simulink model "ATI_NetFT_nano43_PC104"  (R2016a)
settings: Solver=ode3  StartTime=0.0  StopTime=inf  FixedStep=dt  RelTol=1e-3
InitFcn:
  | PSMCMD_DEPENDENCY
  | init_NetFt
  | init_scopes
  | init_udp
  | init_resolved_rates
  | ATI_Init_nano43
  | init_LinIntPathPlan
  | init_force_control
undefined symbols (not defined in the file or in its folder): A, ATI_torque_convert_to_Nmm, filter_coeffs_ATI, filter_coeffs_bias, inv_T, N_ATI, N_bias
libraries: dspswit3 x1, xpcsensoraylib x1, xpcobsoletelib x1, xpcrtudplib x1, slrtlib x1
settings Model: Creator=Andrea  LastModifiedBy=Rashid
settings SolverCC: EnableConcurrentExecution=on
settings DataIOCC: LimitDataPoints=on  SaveFormat=Array  SignalLoggingSaveFormat=ModelDataLogs
settings OptimizationCC: BlockReduction=off  OptimizeBlockIOStorage=off  BufferReuse=off  GlobalBufferReuse=off  ExpressionFolding=off  ExpressionDepthLimit=2147483647  LocalBlockOutputs=off  OptimizeModelRefInitCode=on
settings DebuggingCC: UnderspecifiedInitializationDetection=Classic  MergeDetectMultiDrivingBlocksExec=none  SolverPrmCheckMsg=warning  MultiTaskCondExecSysMsg=warning  MultiTaskRateTransMsg=warning  FcnCallInpInsideContextMsg=UseLocalSettings  StateNameClashWarn=warning
settings HardwareCC: ProdBitPerPointer=32  ProdLargestAtomicFloat=None  ProdWordSize=32  ProdLongLongMode=on  ProdHWDeviceType=Generic->32-bit x86 compatible
settings ModelReferenceCC: PropagateSignalLabelsOutOfModel=off
settings SFSimCC: SimParseCustomCode=off
settings RTWCC: SystemTargetFile=slrtert.tlc  TLCOptions=-aSLRTFTZOFF=1  TemplateMakefile=slrtert_default_tmf  Description=Simulink Real-Time (ERT)  RTWCompilerOptimization=Custom  RTWCustomCompilerOptimizations=/arch=IA32
settings CodeAppCC: CustomSymbolStrType=$N$R$M  InternalIdentifier=Classic
settings SimulinkRealTimeERTCC: TargetFcnLib=ansi_tfl_table_tmw.mat  GenFloatMathFcnCalls=NOT IN USE  TargetLangStandard=C89/C90 (ANSI)  CodeReplacementLibrary=XPC_BLAS  UtilityFuncGeneration=Auto  ERTMultiwordTypeDef=System defined  ERTMultiwordLength=256  MultiwordLength=2048  GenerateFullHeader=on  InferredTypesCompatibility=off  GenerateSampleERTMain=off  GenerateTestInterfaces=off  ModelReferenceCompliant=on  ParMdlRefBuildCompliant=on  CompOptLevelCompliant=on  ConcurrentExecutionCompliant=on  IncludeMdlTerminateFcn=on  GeneratePreprocessorConditionals=Disable all  CombineOutputUpdateFcns=off  CombineSignalStateStructs=off  SuppressErrorStatus=off  ERTFirstTimeCompliant=off  IncludeFileDelimiter=Auto  ERTCustomFileBanners=off  SupportAbsoluteTime=on  LogVarNameModifier=rt_  MatFileLogging=on  MultiInstanceERTCode=off  CodeInterfacePackaging=Nonreusable function  SupportNonFinite=on  SupportComplex=on  PurelyIntegerCode=off  SupportContinuousTime=on  SupportNonInlinedSFcns=on  SupportVariableSizeSignals=off  ParenthesesLevel=Nominal  CastingMode=Nominal  MATLABClassNameForMDSCustomization=xpcAperiodicCustomization  ModelStepFunctionPrototypeControlCompliant=off  CPPClassGenCompliant=off  AutosarCompliant=off  GRTInterface=on  GenerateAllocFcn=off  UseToolchainInfoCompliant=off  GenerateSharedConstants=on  ExtModeTransport=0  ExtModeStaticAlloc=off  ExtModeStaticAllocSize=1000000  ExtModeTesting=off  InlinedParameterPlacement=Hierarchical  TargetOS=BareBoardExample  MultiInstanceErrorCode=Error  RateGroupingCode=on  RootIOFormat=Individual arguments  RTWCAPIRootIO=off  EnableDataOwnership=off  ERTFilePackagingFormat=Modular  PreserveExpressionOrder=off  PreserveIfCondition=off  ConvertIfToSwitch=off  PreserveExternInFcnDecls=on  SuppressUnreachableDefaultCases=off  EnableSignedLeftShifts=on  EnableSignedRightShifts=on  IndentStyle=K&R  IndentSize=2  EnableUserReplacementTypes=off  MaxIdInt32=MAX_int32_T  MinIdInt32=MIN_int32_T  MaxIdUint32=MAX_uint32_T  MaxIdInt16=MAX_int16_T  MinIdInt16=MIN_int16_T  MaxIdUint16=MAX_uint16_T  MaxIdInt8=MAX_int8_T  MinIdInt8=MIN_int8_T  MaxIdUint8=MAX_uint8_T  BooleanTrueId=true  BooleanFalseId=false  MemSecPackage=--- None ---  MemSecDataConstants=Default  MemSecDataIO=Default  MemSecDataInternal=Default  MemSecDataParameters=Default  MemSecFuncInitTerm=Default  MemSecFuncExecute=Default  MemSecFuncSharedUtil=Default  GlobalDataDefinition=Auto  GlobalDataReference=Auto  GenerateASAP2=off  ERTSrcFileBannerTemplate=ert_code_template.cgt  ERTHdrFileBannerTemplate=ert_code_template.cgt  ERTDataSrcFileTemplate=ert_code_template.cgt  ERTDataHdrFileTemplate=ert_code_template.cgt  ERTCustomFileTemplate=example_file_process.tlc  SignalDisplayLevel=10  ParamTuneLevel=10  InitialValueSource=Model  RTWCAPISignals=off  RTWCAPIParams=on  RTWCAPIStates=off  RL32ModeModifier=Real-Time  ExtMode=on  ExtModeMexFile=ext_xpc  ExtModeIntrfLevel=Level2 - Open  ExtModeArmWhenConnect=off  RL32LogTETModifier=on  RL32LogBufSizeModifier=100000  xPCTaskExecutionProfile=off  xPCRL32EventNumber=5000  RL32IRQSourceModifier=Timer  xPCIRQSourceBoard=None/Other  xPCIOIRQSlot=-1  xpcObjCom=off  xPCGenerateASAP2=off  xPCGenerateXML=off  RL32ObjectName=tg  xPCisDownloadable=off  xPCisDefaultEnv=on  xPCisModelTimeout=on  xPCModelTimeoutSecs=5  xpcDblBuff=off  xPCLoadParamSetFile=off  xPCConcurrentTasks=off  xPCEnableSFAnimation=off
settings ConfigComp: CovModelRefEnable=Off

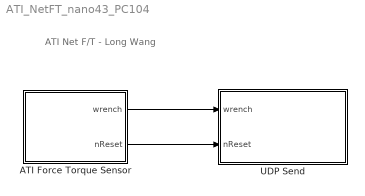
== system ATI_NetFT_nano43_PC104 ==
  note: ATI Net F/T - Long Wang
  ATI Force Torque Sensor : Subsystem
  UDP Send : Subsystem
  wires:
  ATI Force Torque Sensor/1(wrench) -> UDP Send/1(wrench)
  ATI Force Torque Sensor/2(nReset) -> UDP Send/2(nReset)

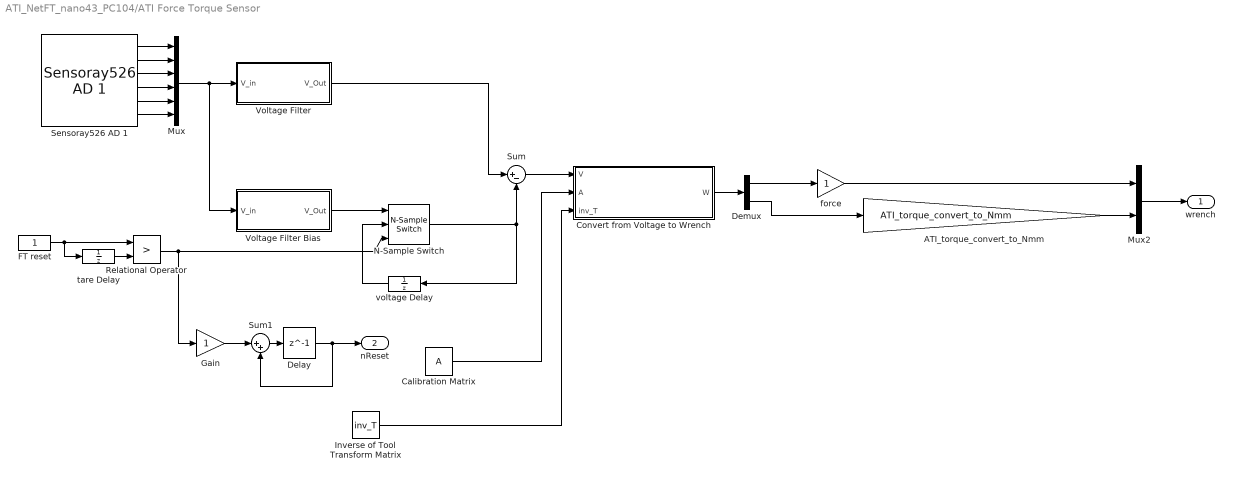
== system ATI_NetFT_nano43_PC104/ATI Force Torque Sensor ==
  ATI_torque_convert_to_Nmm : Gain  Gain=ATI_torque_convert_to_Nmm
  Calibration Matrix : Constant  Value=A
  "Convert from Voltage to Wrench " : MATLAB Function  TreatAsAtomicUnit=on
  Delay : Delay  DelayLength=1  InitialCondition=0
  Demux : Demux  Outputs=2
  FT reset : Constant
  Gain : Gain  OutDataTypeStr=double
  Inverse of Tool Transform Matrix : Constant  Value=inv_T  VectorParams1D=off
  Mux : Mux  Inputs=6
  Mux2 : Mux  Inputs=2
  N-Sample Switch : dspswit3/N-Sample Switch  N=3000  reset=on  TriggerType=Rising edge  Ts=-1
  Relational Operator : RelationalOperator  Operator=>  OutDataTypeStr=boolean
  Sensoray526 AD 1 : xpcsensoraylib/A//D/Sensoray526 AD 1  channel=[1 2 3 4 5 6]  sampletime=.002  baseaddress1=0x2c0  baseaddress2=0
  Sum : Sum  Inputs=|+-
  Sum1 : Sum  Inputs=|++
  Voltage Filter : Subsystem
  Voltage Filter Bias : Subsystem
  force : Gain
  tare Delay : UnitDelay  SampleTime=-1
  voltage Delay : UnitDelay  InitialCondition=zeros(6,1)  SampleTime=-1
  wrench : Outport
  nReset : Outport  Port=2
  wires:
  Sensoray526 AD 1/1 -> Mux/1
  Sensoray526 AD 1/2 -> Mux/2
  Sensoray526 AD 1/3 -> Mux/3
  Sensoray526 AD 1/4 -> Mux/4
  Sensoray526 AD 1/5 -> Mux/5
  Sensoray526 AD 1/6 -> Mux/6
  Calibration Matrix/1 -> "Convert from Voltage to Wrench "/2(A)
  Inverse of Tool Transform Matrix/1 -> "Convert from Voltage to Wrench "/3(inv_T)
  Sum/1 -> "Convert from Voltage to Wrench "/1(V)
  Voltage Filter/1(V_Out) -> Sum/1
  Demux/1 -> force/1
  Demux/2 -> ATI_torque_convert_to_Nmm/1
  ATI_torque_convert_to_Nmm/1 -> Mux2/2
  "Convert from Voltage to Wrench "/1(W) -> Demux/1
  force/1 -> Mux2/1
  Mux2/1 -> wrench/1
  Mux/1 -> Voltage Filter/1(V_in), Voltage Filter Bias/1(V_in)
  FT reset/1 -> Relational Operator/1, tare Delay/1
  tare Delay/1 -> Relational Operator/2
  Voltage Filter Bias/1(V_Out) -> N-Sample Switch/1
  N-Sample Switch/1 -> Sum/2, voltage Delay/1
  voltage Delay/1 -> N-Sample Switch/2
  Delay/1 -> Sum1/2, nReset/1
  Relational Operator/1 -> Gain/1, N-Sample Switch/3
  Sum1/1 -> Delay/1
  Gain/1 -> Sum1/1

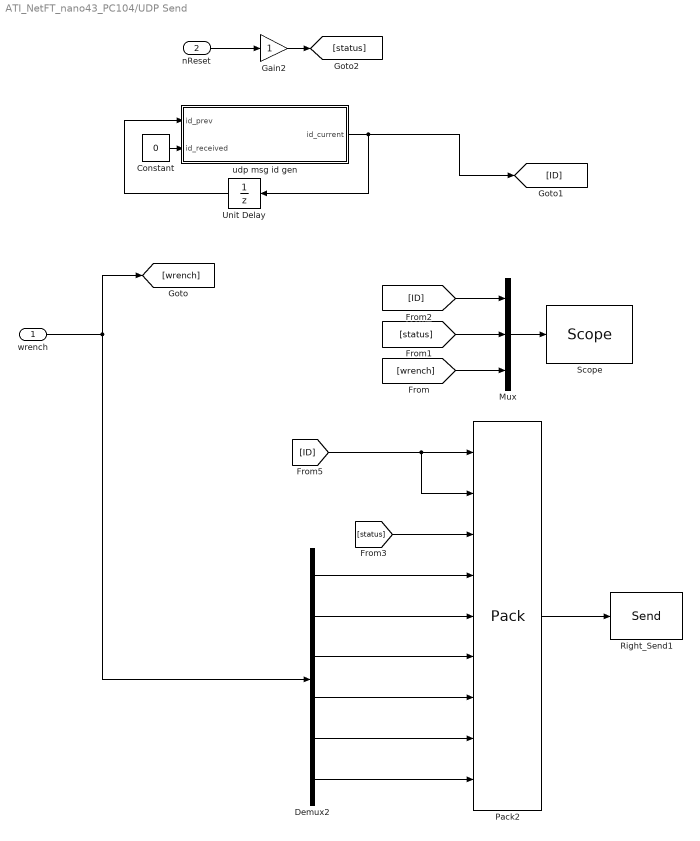
== system ATI_NetFT_nano43_PC104/UDP Send ==
  wrench : Inport
  nReset : Inport  Port=2
  Constant : Constant  Value=0
  Demux2 : Demux  Outputs=6
  Gain2 : Gain
  Mux : Mux  Inputs=[1,1,6]
  Pack2 : xpcobsoletelib/Utilities/Pack   datatypes={'double','double','double','double','double','double','double','double','double'}  byteAlign=1
  Right_Send1 : xpcrtudplib/Legacy UDP/Send   ipAddress=192.168.1.102  ipPort=ATI_NetFt_port  localPort=-1  vblLen=off  sampletime=dt_udp
  "Scope " : slrtlib/Displays and Logging/Scope   scopeno=9  scopetype=Target  autostart=on  viewmode=Numerical  formatstr=Scope_format_socketSentFtMsg  grid=on  ylimits=[0,0]  nosamples=10  noprepostsamples=0  interleave=1  triggermode=FreeRun  triggersignal=1  trigsignalfromport=off  triggerlevel=0.0  triggerslope=Either  triggerscope=1  triggersample=0  filename=data.dat  mode=Lazy  writesize=512  autorestart=off  dynamicfilemode=off  maxwritefilesize=512*1024^2
  Unit Delay : UnitDelay  SampleTime=-1
  udp msg id gen : MATLAB Function  TreatAsAtomicUnit=on
  wires:
  nReset/1 -> Gain2/1
  Unit Delay/1 -> udp msg id gen/1(id_prev)
  Constant/1 -> udp msg id gen/2(id_received)
  udp msg id gen/1(id_current) -> [ID], Unit Delay/1
  Mux/1 -> "Scope "/1
  [wrench] -> Mux/3
  [ID] -> Mux/1
  Gain2/1 -> [status]
  [status] -> Mux/2
  wrench/1 -> Demux2/1, [wrench]
  Demux2/2 -> Pack2/5
  Demux2/4 -> Pack2/7
  Demux2/3 -> Pack2/6
  Demux2/5 -> Pack2/8
  Demux2/6 -> Pack2/9
  Demux2/1 -> Pack2/4
  Pack2/1 -> Right_Send1/1
  [ID] -> Pack2/2, Pack2/1
  [status] -> Pack2/3

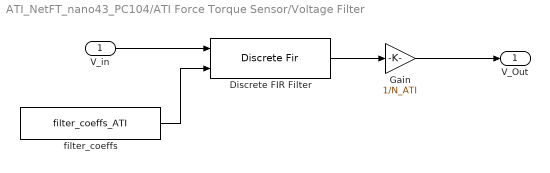
== system ATI_NetFT_nano43_PC104/ATI Force Torque Sensor/Voltage Filter ==
  V_in : Inport
  Discrete FIR Filter : DiscreteFir  CoefSource=Input port  AccumDataTypeStr=Inherit: Same as product output
      settings: InputPortMap=u0,u1
  Gain : Gain  Gain=1/N_ATI
  filter_coeffs : Constant  Value=filter_coeffs_ATI
  V_Out : Outport
  wires:
  V_in/1 -> Discrete FIR Filter/1
  Discrete FIR Filter/1 -> Gain/1
  filter_coeffs/1 -> Discrete FIR Filter/2
  Gain/1 -> V_Out/1

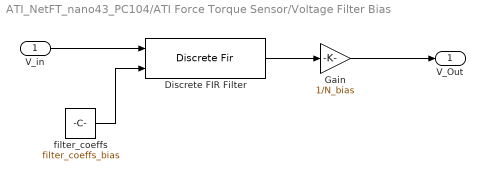
== system ATI_NetFT_nano43_PC104/ATI Force Torque Sensor/Voltage Filter Bias ==
  V_in : Inport
  Discrete FIR Filter : DiscreteFir  CoefSource=Input port  AccumDataTypeStr=Inherit: Same as product output
      settings: InputPortMap=u0,u1
  Gain : Gain  Gain=1/N_bias
  filter_coeffs : Constant  Value=filter_coeffs_bias  SampleTime=-1
  V_Out : Outport
  wires:
  Gain/1 -> V_Out/1
  filter_coeffs/1 -> Discrete FIR Filter/2
  Discrete FIR Filter/1 -> Gain/1
  V_in/1 -> Discrete FIR Filter/1

== matlab function ATI_NetFT_nano43_PC104/ATI Force Torque Sensor/Convert from Voltage to Wrench  ==
  data: V input; W output; A input; inv_T input
function W = Convert_Function(V,A,inv_T)%A_vec,p)

W = inv_T*A*V;

== matlab function ATI_NetFT_nano43_PC104/UDP Send/udp msg id gen ==
  data: id_prev input; id_current output; id_received input
function id_current = MsgIDGen(id_prev,id_received)
%#codegen
%%  Generate message ID
if id_received==1
    id_current = 2;
else
    id_current = id_prev + 1;
end
